simulink model "week4_2016741077_imseyeong_simul"  (R2021a)
settings: Solver=VariableStepAuto  StartTime=0.0  StopTime=1  RelTol=1e-3
values from neighbouring files (symbols this model uses):
  Beq = bm + k*bg + k*B_load    (= 0.003123167094)    [week4_2016741077_imseyeong.m]
  deg_rep = 90    [week4_2016741077_imseyeong.m]
  i_rep = 25    [week4_2016741077_imseyeong.m]
  Jeq = Jm + k*Jg + k*J_load    (= 1.17431082734e-05)    [week4_2016741077_imseyeong.m]
  Ka_cur = 1/Kp_cur    (= 1.20938406605)    [week4_2016741077_imseyeong.m]
  Ka_spd = 1/Kp_spd    (= 0.664805212073)    [week4_2016741077_imseyeong.m]
  Kd_pos = 0.15    [week4_2016741077_imseyeong.m]
  Ke = 68.3*10^-3    (= 0.0683)    [week4_2016741077_imseyeong.m]
  Ki_cur = Ra * Wcc    (= 2211.68122813)    [week4_2016741077_imseyeong.m]
  Ki_spd = 46.660104    [week4_2016741077_imseyeong.m]
  Kp_cur = La * Wcc    (= 0.826867186425)    [week4_2016741077_imseyeong.m]
  Kp_pos = 4.5    [week4_2016741077_imseyeong.m]
  Kp_spd = 1.5042    [week4_2016741077_imseyeong.m]
  Kt = 68.3*10^-3    (= 0.0683)    [week4_2016741077_imseyeong.m]
  La = 0.658*10^-3    (= 0.000658)    [week4_2016741077_imseyeong.m]
  n = 81    [week4_2016741077_imseyeong.m]
  Ra = 1.76    [week4_2016741077_imseyeong.m]
  wm_rep = 5    [week4_2016741077_imseyeong.m]
settings Model: Creator=syl12  LastModifiedBy=syl12

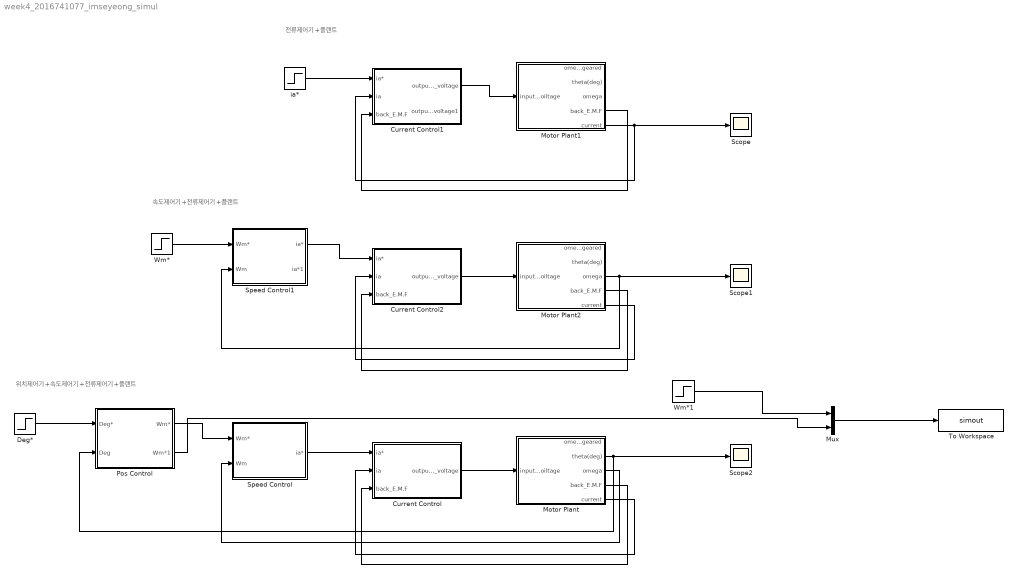
== system week4_2016741077_imseyeong_simul ==
  note: 위치제어기+속도제어기+전류제어기+플랜트
  note: 전류제어기+플랜트
  note: 속도제어기+전류제어기+플랜트
  Current Control : Subsystem
  Current Control1 : Subsystem
  Current Control2 : Subsystem
  Deg* : Step  Time=0  After=deg_rep  SampleTime=0
  Motor Plant : Subsystem
  Motor Plant1 : Subsystem
  Motor Plant2 : Subsystem
  Mux : Mux  Inputs=2
  Pos Control : Subsystem
  Scope : Scope
  Scope1 : Scope
  Scope2 : Scope
  Speed Control : Subsystem
  Speed Control1 : Subsystem
  To Workspace : ToWorkspace  VariableName=simout  SaveFormat=Structure With Time  SampleTime=-1
  Wm* : Step  Time=0  After=wm_rep  SampleTime=0
  Wm*1 : Step  Time=0  After=642.9792964/81  SampleTime=0
  ia* : Step  Time=0  After=i_rep  SampleTime=0
  wires:
  Mux/1 -> To Workspace/1
  Current Control/1(output_voltage) -> Motor Plant/1(input_voiltage)
  Motor Plant/4(back_E.M.F) -> Current Control/3(back_E.M.F)
  Motor Plant/5(current) -> Current Control/2(ia)
  Speed Control/1(ia*) -> Current Control/1(ia*)
  Motor Plant/3(omega) -> Speed Control/2(Wm)
  Pos Control/1(Wm*) -> Speed Control/1(Wm*)
  Motor Plant/2(theta(deg)) -> Scope2/1, Pos Control/2(Deg)
  Deg*/1 -> Pos Control/1(Deg*)
  Motor Plant1/5(current) -> Scope/1, Current Control1/2(ia)
  Motor Plant1/4(back_E.M.F) -> Current Control1/3(back_E.M.F)
  Current Control1/1(output_voltage) -> Motor Plant1/1(input_voiltage)
  ia*/1 -> Current Control1/1(ia*)
  Motor Plant2/3(omega) -> Speed Control1/2(Wm), Scope1/1
  Speed Control1/1(ia*) -> Current Control2/1(ia*)
  Motor Plant2/5(current) -> Current Control2/2(ia)
  Motor Plant2/4(back_E.M.F) -> Current Control2/3(back_E.M.F)
  Current Control2/1(output_voltage) -> Motor Plant2/1(input_voiltage)
  Wm*/1 -> Speed Control1/1(Wm*)
  Wm*1/1 -> Mux/1
  Pos Control/2(Wm*1) -> Mux/2

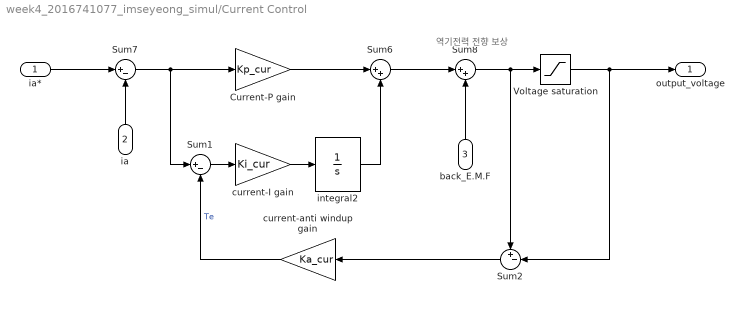
== system week4_2016741077_imseyeong_simul/Current Control ==
  note: 역기전력 전향 보상
  ia* : Inport
  ia : Inport  Port=2
  back_E.M.F : Inport  Port=3
  Current-P gain : Gain  Gain=Kp_cur
  Sum1 : Sum  Inputs=|+-
  Sum2 : Sum  Inputs=+-|
  Sum6 : Sum  Inputs=|++
  Sum7 : Sum  Inputs=|+-
  Sum8 : Sum  Inputs=|++
  Voltage saturation : Saturate  UpperLimit=48  LowerLimit=-48  ZeroCross=off
  current-I gain : Gain  Gain=Ki_cur
  current-anti windup gain : Gain  Gain=Ka_cur
  integral2 : TransferFcn  Denominator=[1 0]
  output_voltage : Outport
  wires:
  Sum6/1 -> Sum8/1
  ia*/1 -> Sum7/1
  integral2/1 -> Sum6/2
  Sum7/1 -> Current-P gain/1, Sum1/1
  Current-P gain/1 -> Sum6/1
  current-I gain/1 -> integral2/1
  back_E.M.F/1 -> Sum8/2
  Voltage saturation/1 -> Sum2/2, output_voltage/1
  Sum8/1 -> Sum2/1, Voltage saturation/1
  ia/1 -> Sum7/2
  Sum1/1 -> current-I gain/1
  current-anti windup gain/1 -> Sum1/2  "Te"
  Sum2/1 -> current-anti windup gain/1

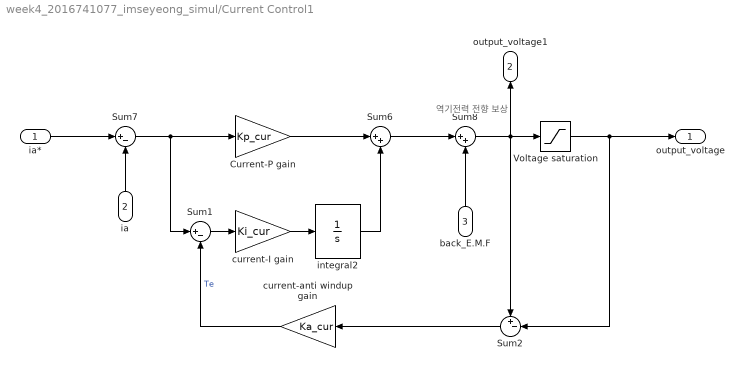
== system week4_2016741077_imseyeong_simul/Current Control1 ==
  note: 역기전력 전향 보상
  ia* : Inport
  ia : Inport  Port=2
  back_E.M.F : Inport  Port=3
  Current-P gain : Gain  Gain=Kp_cur
  Sum1 : Sum  Inputs=|+-
  Sum2 : Sum  Inputs=+-|
  Sum6 : Sum  Inputs=|++
  Sum7 : Sum  Inputs=|+-
  Sum8 : Sum  Inputs=|++
  Voltage saturation : Saturate  UpperLimit=48  LowerLimit=-48  ZeroCross=off
  current-I gain : Gain  Gain=Ki_cur
  current-anti windup gain : Gain  Gain=Ka_cur
  integral2 : TransferFcn  Denominator=[1 0]
  output_voltage : Outport
  output_voltage1 : Outport  Port=2
  wires:
  Sum2/1 -> current-anti windup gain/1
  current-anti windup gain/1 -> Sum1/2  "Te"
  Sum1/1 -> current-I gain/1
  ia/1 -> Sum7/2
  Sum8/1 -> Voltage saturation/1, Sum2/1, output_voltage1/1
  Voltage saturation/1 -> output_voltage/1, Sum2/2
  back_E.M.F/1 -> Sum8/2
  current-I gain/1 -> integral2/1
  Current-P gain/1 -> Sum6/1
  Sum7/1 -> Sum1/1, Current-P gain/1
  integral2/1 -> Sum6/2
  ia*/1 -> Sum7/1
  Sum6/1 -> Sum8/1

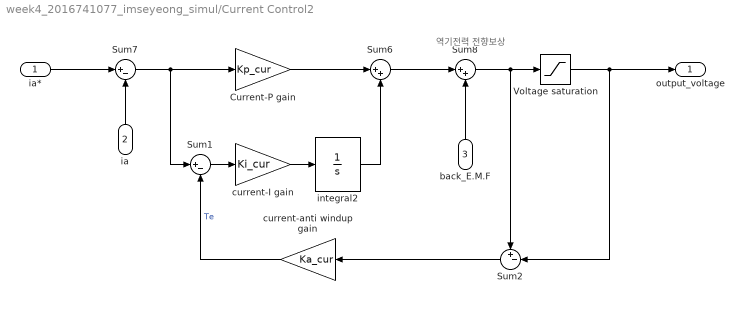
== system week4_2016741077_imseyeong_simul/Current Control2 ==
  note: 역기전력 전향보상
  ia* : Inport
  ia : Inport  Port=2
  back_E.M.F : Inport  Port=3
  Current-P gain : Gain  Gain=Kp_cur
  Sum1 : Sum  Inputs=|+-
  Sum2 : Sum  Inputs=+-|
  Sum6 : Sum  Inputs=|++
  Sum7 : Sum  Inputs=|+-
  Sum8 : Sum  Inputs=|++
  Voltage saturation : Saturate  UpperLimit=48  LowerLimit=-48  ZeroCross=off
  current-I gain : Gain  Gain=Ki_cur
  current-anti windup gain : Gain  Gain=Ka_cur
  integral2 : TransferFcn  Denominator=[1 0]
  output_voltage : Outport
  wires:
  Sum2/1 -> current-anti windup gain/1
  current-anti windup gain/1 -> Sum1/2  "Te"
  Sum1/1 -> current-I gain/1
  ia/1 -> Sum7/2
  Sum8/1 -> Voltage saturation/1, Sum2/1
  Voltage saturation/1 -> output_voltage/1, Sum2/2
  back_E.M.F/1 -> Sum8/2
  current-I gain/1 -> integral2/1
  Current-P gain/1 -> Sum6/1
  Sum7/1 -> Sum1/1, Current-P gain/1
  integral2/1 -> Sum6/2
  ia*/1 -> Sum7/1
  Sum6/1 -> Sum8/1

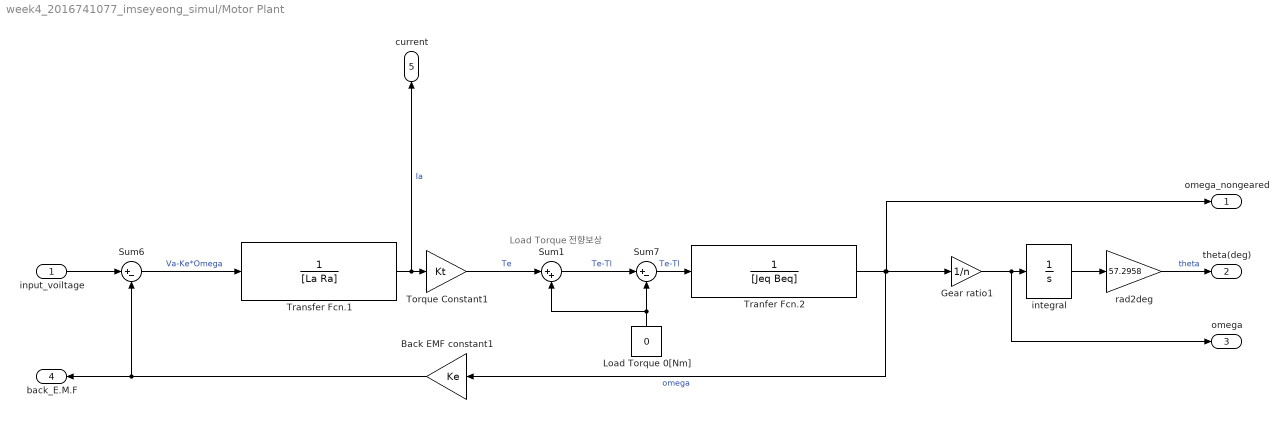
== system week4_2016741077_imseyeong_simul/Motor Plant ==
  note: Load Torque 전향보상
  input_voiltage : Inport
  Back EMF constant1 : Gain  Gain=Ke
  Gear ratio1 : Gain  Gain=1/n
  Load Torque 0[Nm] : Constant  Value=0
  Sum1 : Sum  Inputs=|++
  Sum6 : Sum  Inputs=|+-
  Sum7 : Sum  Inputs=|+-
  Torque Constant1 : Gain  Gain=Kt
  Tranfer Fcn.2 : TransferFcn  Denominator=[Jeq Beq]
  Transfer Fcn.1 : TransferFcn  Denominator=[La Ra]
  integral : TransferFcn  Denominator=[1 0]
  rad2deg : Gain  Gain=57.2958
  omega_nongeared : Outport
  theta(deg) : Outport  Port=2
  omega : Outport  Port=3
  back_E.M.F : Outport  Port=4
  current : Outport  Port=5
  wires:
  Sum6/1 -> Transfer Fcn.1/1  "Va-Ke*Omega"
  Tranfer Fcn.2/1 -> omega_nongeared/1, Gear ratio1/1, Back EMF constant1/1  "omega"
  Sum7/1 -> Tranfer Fcn.2/1  "Te-Tl"
  Back EMF constant1/1 -> back_E.M.F/1, Sum6/2
  input_voiltage/1 -> Sum6/1
  Transfer Fcn.1/1 -> Torque Constant1/1, current/1  "Ia"
  integral/1 -> rad2deg/1
  rad2deg/1 -> theta(deg)/1  "theta"
  Gear ratio1/1 -> omega/1, integral/1
  Torque Constant1/1 -> Sum1/1  "Te"
  Sum1/1 -> Sum7/1  "Te-Tl"
  Load Torque 0[Nm]/1 -> Sum1/2, Sum7/2

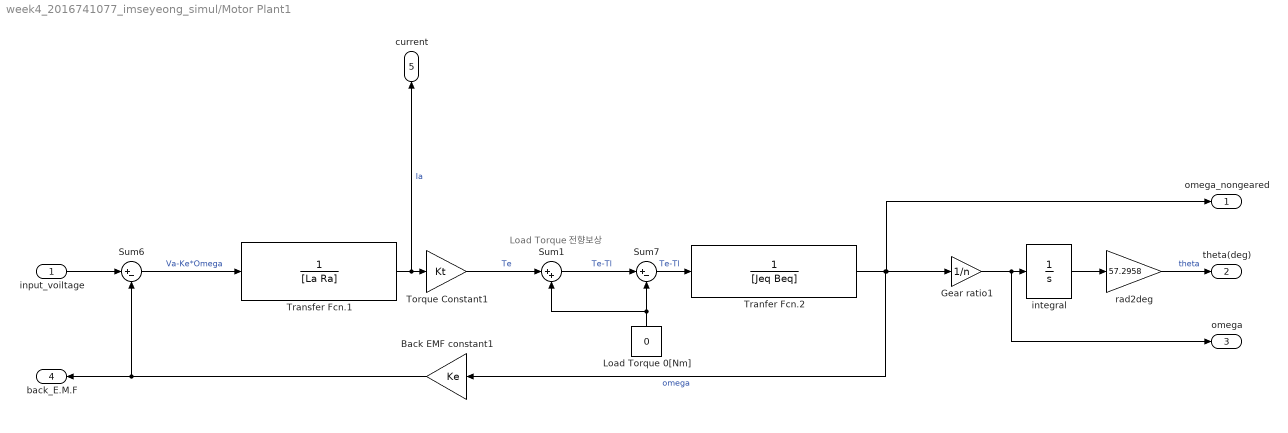
== system week4_2016741077_imseyeong_simul/Motor Plant1 ==
  note: Load Torque 전향보상
  input_voiltage : Inport
  Back EMF constant1 : Gain  Gain=Ke
  Gear ratio1 : Gain  Gain=1/n
  Load Torque 0[Nm] : Constant  Value=0
  Sum1 : Sum  Inputs=|++
  Sum6 : Sum  Inputs=|+-
  Sum7 : Sum  Inputs=|+-
  Torque Constant1 : Gain  Gain=Kt
  Tranfer Fcn.2 : TransferFcn  Denominator=[Jeq Beq]
  Transfer Fcn.1 : TransferFcn  Denominator=[La Ra]
  integral : TransferFcn  Denominator=[1 0]
  rad2deg : Gain  Gain=57.2958
  omega_nongeared : Outport
  theta(deg) : Outport  Port=2
  omega : Outport  Port=3
  back_E.M.F : Outport  Port=4
  current : Outport  Port=5
  wires:
  Load Torque 0[Nm]/1 -> Sum7/2, Sum1/2
  Sum1/1 -> Sum7/1  "Te-Tl"
  Torque Constant1/1 -> Sum1/1  "Te"
  Gear ratio1/1 -> integral/1, omega/1
  rad2deg/1 -> theta(deg)/1  "theta"
  integral/1 -> rad2deg/1
  Transfer Fcn.1/1 -> current/1, Torque Constant1/1  "Ia"
  input_voiltage/1 -> Sum6/1
  Back EMF constant1/1 -> Sum6/2, back_E.M.F/1
  Sum7/1 -> Tranfer Fcn.2/1  "Te-Tl"
  Tranfer Fcn.2/1 -> Back EMF constant1/1, Gear ratio1/1, omega_nongeared/1  "omega"
  Sum6/1 -> Transfer Fcn.1/1  "Va-Ke*Omega"

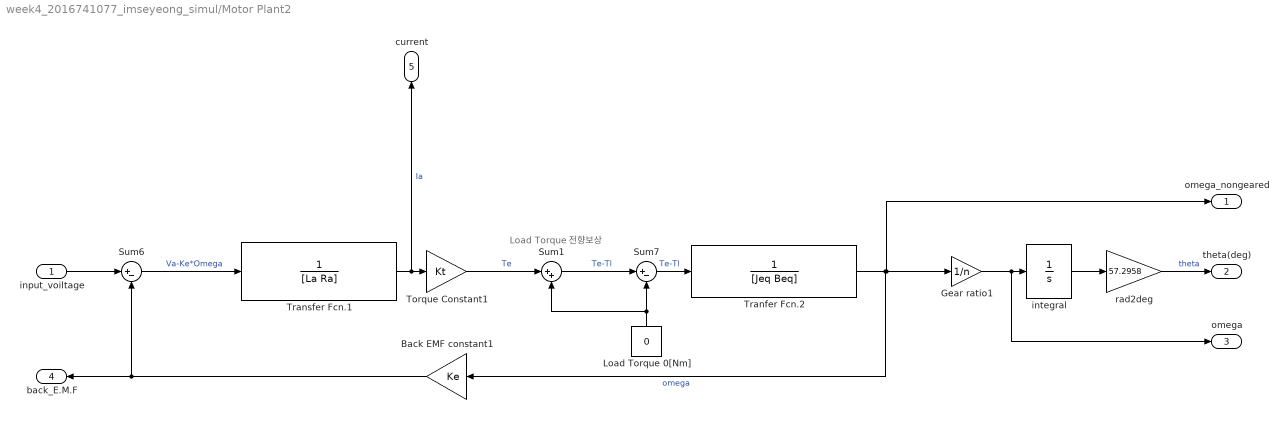
== system week4_2016741077_imseyeong_simul/Motor Plant2 ==
  note: Load Torque 전향보상
  input_voiltage : Inport
  Back EMF constant1 : Gain  Gain=Ke
  Gear ratio1 : Gain  Gain=1/n
  Load Torque 0[Nm] : Constant  Value=0
  Sum1 : Sum  Inputs=|++
  Sum6 : Sum  Inputs=|+-
  Sum7 : Sum  Inputs=|+-
  Torque Constant1 : Gain  Gain=Kt
  Tranfer Fcn.2 : TransferFcn  Denominator=[Jeq Beq]
  Transfer Fcn.1 : TransferFcn  Denominator=[La Ra]
  integral : TransferFcn  Denominator=[1 0]
  rad2deg : Gain  Gain=57.2958
  omega_nongeared : Outport
  theta(deg) : Outport  Port=2
  omega : Outport  Port=3
  back_E.M.F : Outport  Port=4
  current : Outport  Port=5
  wires:
  Load Torque 0[Nm]/1 -> Sum7/2, Sum1/2
  Sum1/1 -> Sum7/1  "Te-Tl"
  Torque Constant1/1 -> Sum1/1  "Te"
  Gear ratio1/1 -> integral/1, omega/1
  rad2deg/1 -> theta(deg)/1  "theta"
  integral/1 -> rad2deg/1
  Transfer Fcn.1/1 -> current/1, Torque Constant1/1  "Ia"
  input_voiltage/1 -> Sum6/1
  Back EMF constant1/1 -> Sum6/2, back_E.M.F/1
  Sum7/1 -> Tranfer Fcn.2/1  "Te-Tl"
  Tranfer Fcn.2/1 -> Back EMF constant1/1, Gear ratio1/1, omega_nongeared/1  "omega"
  Sum6/1 -> Transfer Fcn.1/1  "Va-Ke*Omega"

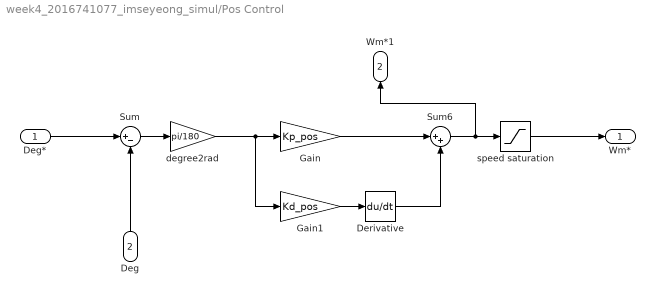
== system week4_2016741077_imseyeong_simul/Pos Control ==
  Deg* : Inport
  Deg : Inport  Port=2
  Derivative : Derivative
  Gain : Gain  Gain=Kp_pos
  Gain1 : Gain  Gain=Kd_pos
  Sum : Sum  Inputs=|+-
  Sum6 : Sum  Inputs=|++
  degree2rad : Gain  Gain=pi/180
  speed saturation : Saturate  UpperLimit=642.9792964/81  LowerLimit=-642.9792964/81
  Wm* : Outport
  Wm*1 : Outport  Port=2
  wires:
  Derivative/1 -> Sum6/2
  Deg*/1 -> Sum/1
  speed saturation/1 -> Wm*/1
  Gain/1 -> Sum6/1
  Sum6/1 -> speed saturation/1, Wm*1/1
  Deg/1 -> Sum/2
  Gain1/1 -> Derivative/1
  Sum/1 -> degree2rad/1
  degree2rad/1 -> Gain1/1, Gain/1

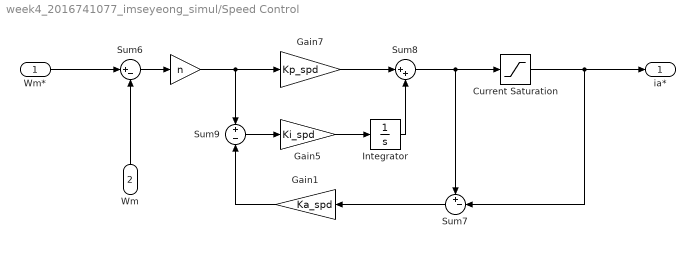
== system week4_2016741077_imseyeong_simul/Speed Control ==
  Wm* : Inport
  Wm : Inport  Port=2
  " " : Gain  Gain=n
  Current Saturation : Saturate  UpperLimit=27.3  LowerLimit=-27.3  ZeroCross=off
  Gain1 : Gain  Gain=Ka_spd
  Gain5 : Gain  Gain=Ki_spd
  Gain7 : Gain  Gain=Kp_spd
  Integrator : Integrator
  Sum6 : Sum  Inputs=|+-
  Sum7 : Sum  Inputs=+-|
  Sum8 : Sum  Inputs=|++
  Sum9 : Sum  Inputs=+|-
  ia* : Outport
  wires:
  Gain5/1 -> Integrator/1
  Sum8/1 -> Current Saturation/1, Sum7/1
  Current Saturation/1 -> Sum7/2, ia*/1
  Wm/1 -> Sum6/2
  Gain1/1 -> Sum9/2
  Integrator/1 -> Sum8/2
  " "/1 -> Gain7/1, Sum9/1
  Sum6/1 -> " "/1
  Sum7/1 -> Gain1/1
  Gain7/1 -> Sum8/1
  Wm*/1 -> Sum6/1
  Sum9/1 -> Gain5/1

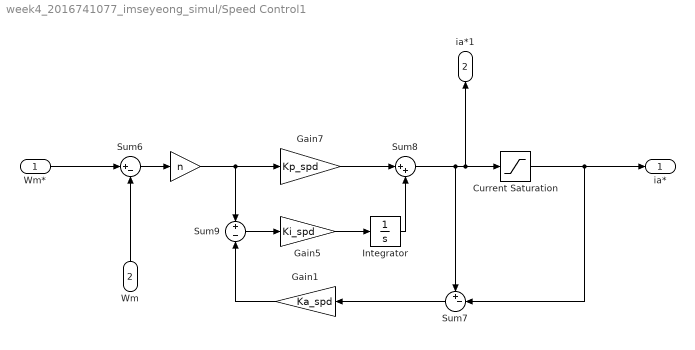
== system week4_2016741077_imseyeong_simul/Speed Control1 ==
  Wm* : Inport
  Wm : Inport  Port=2
  " " : Gain  Gain=n
  Current Saturation : Saturate  UpperLimit=27.3  LowerLimit=-27.3  ZeroCross=off
  Gain1 : Gain  Gain=Ka_spd
  Gain5 : Gain  Gain=Ki_spd
  Gain7 : Gain  Gain=Kp_spd
  Integrator : Integrator
  Sum6 : Sum  Inputs=|+-
  Sum7 : Sum  Inputs=+-|
  Sum8 : Sum  Inputs=|++
  Sum9 : Sum  Inputs=+|-
  ia* : Outport
  ia*1 : Outport  Port=2
  wires:
  Sum9/1 -> Gain5/1
  Wm*/1 -> Sum6/1
  Gain7/1 -> Sum8/1
  Sum7/1 -> Gain1/1
  Sum6/1 -> " "/1
  " "/1 -> Sum9/1, Gain7/1
  Integrator/1 -> Sum8/2
  Gain1/1 -> Sum9/2
  Wm/1 -> Sum6/2
  Current Saturation/1 -> ia*/1, Sum7/2
  Sum8/1 -> Sum7/1, ia*1/1, Current Saturation/1
  Gain5/1 -> Integrator/1
